simulink model "StateSpaceNew1"  (R2023b)
settings: Solver=VariableStepAuto  StartTime=0.0  StopTime=1000  RelTol=1e-3
values from neighbouring files (symbols this model uses):
  designSys = sys0    [LQR2States.m]    (also in LQR2StatesWithDisturb.m; LQR2StatesWithDisturbRecirc.m = sys100)
  L = place(A', -C', observer_poles)'    [IntegralActionWithObs.m]    (also in LQR1.m = place(A_new', C_new', p)'; LQR2States.m = place(designSys.A', designSys.C', observer_poles)'; LQR2StatesWithDisturb.m = place(designSys.A', designSys.C', observer_poles)'; LQR2StatesWithDisturbRecirc.m = place(designSys.A', specialC', observer_poles)')
  N_ref = N*v    [LQR2States.m]    (also in LQR2StatesWithDisturb.m; LQR2StatesWithDisturbRecirc.m)
  u_ref = [zeros(numOutputs, 200), repmat(ref, 1, 800)]    [LQR2States.m]    (also in LQR2StatesWithDisturb.m; LQR2StatesWithDisturbRecirc.m)
undefined symbols (not defined in the file or in its folder): K
settings Model: Creator=jeppe  LastModifiedBy=helen
settings SolverCC: AutoInsertRateTranBlk=on

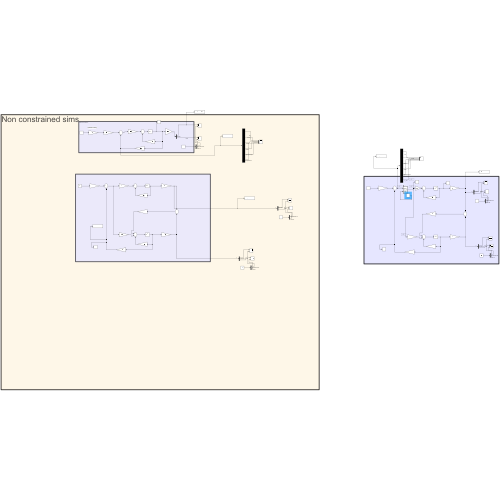
[thumbnail: Simulink's stored preview of the top-level diagram]
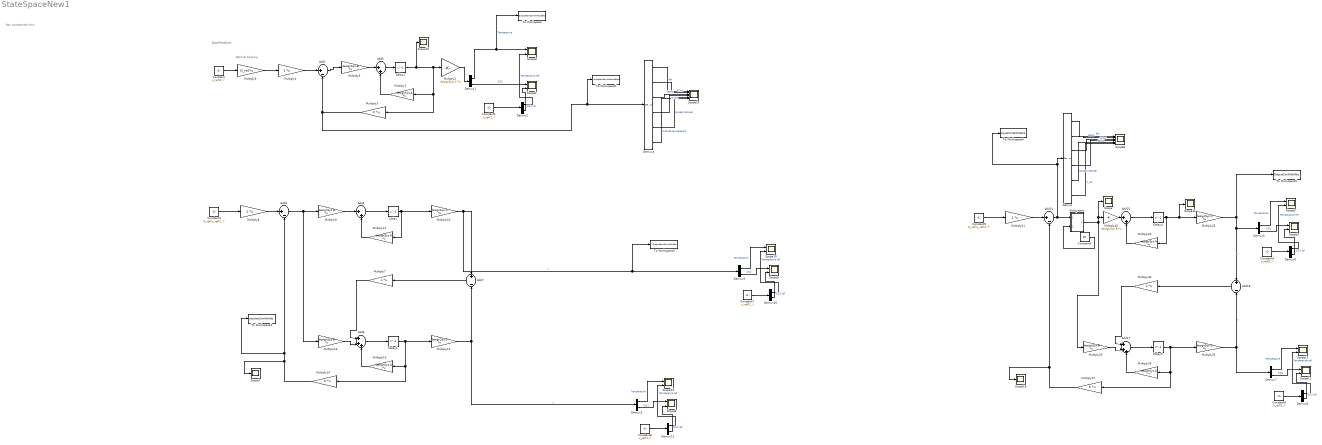
== system StateSpaceNew1 ==
  note: Optimal tracking
  note: Non constrained sims
  note: StateFeedback
  Add1 : Sum  Inputs=|+-
  Add14 : Sum  Inputs=|+-
  Add15 : Sum  Inputs=|++
  Add17 : Sum  Inputs=|+++
  Add18 : Sum  Inputs=+|-
  Add3 : Sum  Inputs=|+-
  Add4 : Sum  Inputs=|++
  Add5 : Sum  Inputs=|++
  Add6 : Sum  Inputs=|+++
  Add7 : Sum  Inputs=+|-
  Constant : Constant  Value=u_ref(2,:)'
  Constant{1,4,6..8} (5 alike) : Constant  Value=u_ref(2,:)
  Constant2 : Constant  Value=N_ref*u_ref(2,:)'
  Constant3 : Constant  Value=15
  Constant5 : Constant  Value=N_ref*u_ref(2,:)'
  Delay{,1..2,4..5} (5 alike) : Delay  DelayLength=1
  Demux : Demux  Outputs=6
  Demux{1..3,5..11} (10 alike) : Demux  Outputs=2
  Demux4 : Demux  Outputs=6
  Multiply{1,11,13,24,26} (5 alike) : Gain  Gain=designSys.A  Multiplication=Matrix(K*u)
  Multiply{2,10,12,23,25} (5 alike) : Gain  Gain=designSys.C  Multiplication=Matrix(K*u)
  Multiply14 : Gain  Gain=K  Multiplication=Matrix(K*u)
  Multiply{5,9,16,29,42} (5 alike) : Gain  Gain=designSys.B  Multiplication=Matrix(K*u)
  Multiply27 : Gain  Gain=K  Multiplication=Matrix(K*u)
  Multiply3 : Gain  Gain=K  Multiplication=Matrix(K*u)
  Multiply4 : Gain  Multiplication=Matrix(K*u)
  Multiply40 : Gain  Gain=L  Multiplication=Matrix(K*u)
  Multiply41 : Gain  Multiplication=Matrix(K*u)
  Multiply6 : Gain  Gain=N_ref  Multiplication=Matrix(K*u)
  Multiply7 : Gain  Gain=L  Multiplication=Matrix(K*u)
  Multiply8 : Gain  Multiplication=Matrix(K*u)
  Scope{,7,15..16,18} (5 alike) : Scope
  Scope{1,3..6,9..13} (10 alike) : Scope  NumInputPorts=2
  Scope14 : Scope  NumInputPorts=6
  Scope8 : Scope  NumInputPorts=6
  Subsystem : Subsystem  TreatAsAtomicUnit=on  ScheduleAs=Periodic partition  PartitionName=Subsystem  SystemSampleTime=15
  To Workspace : ToWorkspace  VariableName=OutputNonConWithoutObs  SampleTime=-1
  To Workspace1 : ToWorkspace  VariableName=InputNonConWithoutObs1  SampleTime=-1
  To Workspace2 : ToWorkspace  VariableName=OutputNonConWithObs  SampleTime=-1
  To Workspace3 : ToWorkspace  VariableName=InputNonConWithObs  SampleTime=-1
  To Workspace4 : ToWorkspace  VariableName=InputConWithObs1  SampleTime=-1
  To Workspace5 : ToWorkspace  VariableName=OutputConWithObs  SampleTime=-1
  wires:
  Demux1/1 -> To Workspace/1, Scope4/1  "Temperature"
  Demux1/2 -> Scope1/1  "CO2"
  Multiply2/1 -> Demux1/1  "y"
  Constant2/1 -> Multiply8/1
  Multiply8/1 -> Add3/1
  Multiply9/1 -> Add4/1
  Add4/1 -> Delay/1
  Multiply11/1 -> Add4/2
  Delay/1 -> Multiply11/1, Multiply10/1
  Add6/1 -> Delay1/1
  Multiply14/1 -> To Workspace3/1, Add3/2, Scope7/1
  Add3/1 -> Multiply16/1, Multiply9/1
  Delay1/1 -> Multiply12/1, Multiply14/1, Multiply13/1
  Add7/1 -> Multiply7/1
  Multiply7/1 -> Add6/1
  Multiply13/1 -> Add6/3
  Multiply16/1 -> Add6/2
  Add15/1 -> Delay4/1
  Constant5/1 -> Multiply41/1
  Add18/1 -> Multiply40/1
  Multiply24/1 -> Add15/2
  Multiply41/1 -> Add14/1
  Delay4/1 -> Multiply24/1, Scope16/1, Multiply23/1
  Multiply40/1 -> Add17/1
  Multiply29/1 -> Add17/2
  Multiply27/1 -> Add14/2, Scope18/1
  Add17/1 -> Delay5/1
  Delay5/1 -> Multiply25/1, Multiply27/1, Multiply26/1
  Multiply26/1 -> Add17/3
  Constant3/1 -> Subsystem/2(T_AO)
  Multiply42/1 -> Add15/1
  Subsystem/1(Out1) -> Scope/1, Multiply42/1, Multiply29/1
  Constant1/1 -> Demux2/1
  Demux2/1 -> Scope4/2  "Temperature ref"
  Demux2/2 -> Scope1/2  "CO2 ref"
  Demux5/2 -> Scope3/1  "CO2"
  Demux5/1 -> Scope5/1  "Temperature"
  Demux6/1 -> Scope5/2  "Temperature ref"
  Constant4/1 -> Demux6/1
  Multiply23/1 -> Demux5/1, Add18/1, To Workspace5/1  "y"
  Demux6/2 -> Scope3/2  "CO2 ref"
  Demux7/2 -> Scope11/1  "CO2"
  Demux7/1 -> Scope12/1  "Temperature"
  Demux8/1 -> Scope12/2  "Temperature ref"
  Constant6/1 -> Demux8/1
  Multiply25/1 -> Demux7/1, Add18/2  "y"
  Demux8/2 -> Scope11/2  "CO2 ref"
  Demux9/2 -> Scope9/1  "CO2"
  Demux9/1 -> Scope10/1  "Temperature"
  Demux10/1 -> Scope10/2  "Temperature ref"
  Constant7/1 -> Demux10/1
  Multiply10/1 -> To Workspace2/1, Demux9/1, Add7/1  "y"
  Demux10/2 -> Scope9/2  "CO2 ref"
  Demux3/2 -> Scope6/1  "CO2"
  Demux3/1 -> Scope13/1  "Temperature"
  Demux11/1 -> Scope13/2  "Temperature ref"
  Constant8/1 -> Demux11/1
  Multiply12/1 -> Add7/2, Demux3/1  "y"
  Demux11/2 -> Scope6/2  "CO2 ref"
  Demux/1 -> Scope8/1  "fan"
  Demux/2 -> Scope8/2  "ECH1"
  Demux/4 -> Scope8/4  "HVAC"
  Demux/5 -> Scope8/5  "Bypass damper"
  Demux4/4 -> Scope14/4  "HVAC"
  Demux4/5 -> Scope14/5  "Bypass damper"
  Demux4/1 -> Scope14/1  "fan"
  Multiply3/1 -> Add1/2, To Workspace1/1, Demux4/1
  Demux4/3 -> Scope14/3  "ECH2"
  Demux4/2 -> Scope14/2  "ECH1"
  Demux4/6 -> Scope14/6  "Outside temperature"
  Add14/1 -> To Workspace4/1, Demux/1, Subsystem/1(signals)
  Demux/3 -> Scope8/3  "ECH2"
  Demux/6 -> Scope8/6  "T_AO"
  Add5/1 -> Delay2/1
  Multiply1/1 -> Add5/2
  Multiply5/1 -> Add5/1
  Add1/1 -> Multiply5/1
  Multiply6/1 -> Multiply4/1
  Multiply4/1 -> Add1/1
  Delay2/1 -> Scope15/1, Multiply3/1, Multiply1/1, Multiply2/1
  Constant/1 -> Multiply6/1

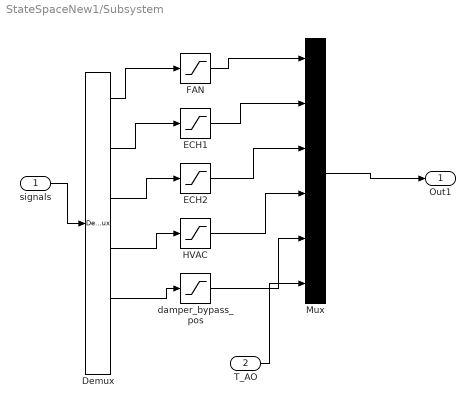
== system StateSpaceNew1/Subsystem ==
  signals : Inport
  T_AO : Inport  Port=2
  Demux : Demux  Outputs=6
  ECH1 : Saturate  UpperLimit=100  LowerLimit=0
  ECH2 : Saturate  UpperLimit=100  LowerLimit=0
  FAN : Saturate  UpperLimit=100  LowerLimit=0
  HVAC : Saturate  UpperLimit=100  LowerLimit=-100
  Mux : Mux  Inputs=6
  damper_bypass_pos : Saturate  UpperLimit=100  LowerLimit=0
  Out1 : Outport
  wires:
  signals/1 -> Demux/1
  Demux/1 -> FAN/1
  Demux/2 -> ECH1/1
  Demux/3 -> ECH2/1
  Demux/4 -> HVAC/1
  Demux/5 -> damper_bypass_pos/1
  FAN/1 -> Mux/1
  ECH1/1 -> Mux/2
  ECH2/1 -> Mux/3
  HVAC/1 -> Mux/4
  damper_bypass_pos/1 -> Mux/5
  T_AO/1 -> Mux/6
  Mux/1 -> Out1/1
